simulink model "case5"  (R2024b)
settings: Solver=FixedStepAuto  StartTime=0  StopTime=1  FixedStep=1e-7  RelTol=1e-3
values from neighbouring files (symbols this model uses):
  SG_D_1_D = 0.01056    [IEEE9_case_parameters.m]    (also in case1_parameters.m; case2_parameters.m; case3_parameters.m; case4_parameters.m)
  SG_D_1_EnableSaturation = 0    [IEEE9_case_parameters.m]    (also in case1_parameters.m; case2_parameters.m; case3_parameters.m; case4_parameters.m)
  SG_D_1_f0 = 60    [IEEE9_case_parameters.m]    (also in case1_parameters.m; case2_parameters.m; case3_parameters.m; case4_parameters.m)
  SG_D_1_H = 7.5    [IEEE9_case_parameters.m]    (also in case1_parameters.m; case2_parameters.m; case3_parameters.m; case4_parameters.m)
  SG_D_1_K_A = 20    [IEEE9_case_parameters.m]    (also in case1_parameters.m; case2_parameters.m; case3_parameters.m; case4_parameters.m)
  SG_D_1_K_E = 1.000000e+1    (= 10)    [IEEE9_case_parameters.m]    (also in case1_parameters.m; case2_parameters.m; case3_parameters.m; case4_parameters.m)
  SG_D_1_K_F = 2.363    [IEEE9_case_parameters.m]    (also in case1_parameters.m; case2_parameters.m; case3_parameters.m; case4_parameters.m)
  SG_D_1_K_s = 0.5    [IEEE9_case_parameters.m]    (also in case1_parameters.m = 5; case2_parameters.m = 5; case3_parameters.m = 5; case4_parameters.m = 5)
  SG_D_1_R_a = 0.001088    [IEEE9_case_parameters.m]    (also in case1_parameters.m; case2_parameters.m; case3_parameters.m; case4_parameters.m)
  SG_D_1_S_A = 1    [IEEE9_case_parameters.m]    (also in case1_parameters.m; case2_parameters.m; case3_parameters.m; case4_parameters.m)
  SG_D_1_S_B = 0.103    [IEEE9_case_parameters.m]    (also in case1_parameters.m; case2_parameters.m; case3_parameters.m; case4_parameters.m)
  SG_D_1_S_N = 10.659857    [IEEE9_case_parameters.m]    (also in case1_parameters.m; case2_parameters.m; case3_parameters.m; case4_parameters.m)
  SG_D_1_SpeedPara = 200    [IEEE9_case_parameters.m]    (also in case1_parameters.m; case2_parameters.m; case3_parameters.m; case4_parameters.m)
  SG_D_1_T_0 = 0.720173    [IEEE9_case_parameters.m]    (also in case1_parameters.m = 0.755522; case2_parameters.m = 0.808931; case3_parameters.m = 0.869402; case4_parameters.m = 0.729316)
  SG_D_1_T_1 = 0.3    [IEEE9_case_parameters.m]    (also in case1_parameters.m; case2_parameters.m; case3_parameters.m; case4_parameters.m)
  SG_D_1_T_2 = 0.05    [IEEE9_case_parameters.m]    (also in case1_parameters.m; case2_parameters.m; case3_parameters.m; case4_parameters.m)
  SG_D_1_T_3 = 0.02    [IEEE9_case_parameters.m]    (also in case1_parameters.m; case2_parameters.m; case3_parameters.m; case4_parameters.m)
  SG_D_1_T_4 = 0.005    [IEEE9_case_parameters.m]    (also in case1_parameters.m; case2_parameters.m; case3_parameters.m; case4_parameters.m)
  SG_D_1_T_A = 0.02    [IEEE9_case_parameters.m]    (also in case1_parameters.m; case2_parameters.m; case3_parameters.m; case4_parameters.m)
  SG_D_1_T_dd = 8.000000e+0    (= 8)    [IEEE9_case_parameters.m]    (also in case1_parameters.m; case2_parameters.m; case3_parameters.m; case4_parameters.m)
  SG_D_1_T_ddd = 0.04    [IEEE9_case_parameters.m]    (also in case1_parameters.m; case2_parameters.m; case3_parameters.m; case4_parameters.m)
  SG_D_1_T_E = 0.314    [IEEE9_case_parameters.m]    (also in case1_parameters.m; case2_parameters.m; case3_parameters.m; case4_parameters.m)
  SG_D_1_T_F = 0.35    [IEEE9_case_parameters.m]    (also in case1_parameters.m; case2_parameters.m; case3_parameters.m; case4_parameters.m)
  SG_D_1_T_qd = 0.8    [IEEE9_case_parameters.m]    (also in case1_parameters.m; case2_parameters.m; case3_parameters.m; case4_parameters.m)
  SG_D_1_T_qdd = 0.02    [IEEE9_case_parameters.m]    (also in case1_parameters.m; case2_parameters.m; case3_parameters.m; case4_parameters.m)
  SG_D_1_T_speed = 0.1    [IEEE9_case_parameters.m]    (also in case1_parameters.m = 200; case2_parameters.m = 200; case3_parameters.m = 200; case4_parameters.m = 200)
  SG_D_1_T_w = 0.5    [IEEE9_case_parameters.m]    (also in case1_parameters.m; case2_parameters.m; case3_parameters.m; case4_parameters.m)
  SG_D_1_V_ref = 1.990276    [IEEE9_case_parameters.m]    (also in case1_parameters.m = 2.042296; case2_parameters.m = 2.051388; case3_parameters.m = 2.089584; case4_parameters.m = 2.01845)
  SG_D_1_w_ref = 376.991118    [IEEE9_case_parameters.m]    (also in case1_parameters.m; case2_parameters.m; case3_parameters.m; case4_parameters.m)
  SG_D_1_wb = 6.000000e+1    (= 60)    [IEEE9_case_parameters.m]    (also in case1_parameters.m; case2_parameters.m; case3_parameters.m; case4_parameters.m)
  SG_D_1_x_d = 1.9    [IEEE9_case_parameters.m]    (also in case1_parameters.m; case2_parameters.m; case3_parameters.m; case4_parameters.m)
  SG_D_1_x_dd = 0.302    [IEEE9_case_parameters.m]    (also in case1_parameters.m; case2_parameters.m; case3_parameters.m; case4_parameters.m)
  SG_D_1_x_ddd = 0.204    [IEEE9_case_parameters.m]    (also in case1_parameters.m; case2_parameters.m; case3_parameters.m; case4_parameters.m)
  SG_D_1_x_l = 0.05    [IEEE9_case_parameters.m]    (also in case1_parameters.m; case2_parameters.m; case3_parameters.m; case4_parameters.m)
  SG_D_1_x_q = 1.3    [IEEE9_case_parameters.m]    (also in case1_parameters.m; case2_parameters.m; case3_parameters.m; case4_parameters.m)
  SG_D_1_x_qd = 0.5    [IEEE9_case_parameters.m]    (also in case1_parameters.m; case2_parameters.m; case3_parameters.m; case4_parameters.m)
  SG_D_1_x_qdd = 0.3    [IEEE9_case_parameters.m]    (also in case1_parameters.m; case2_parameters.m; case3_parameters.m; case4_parameters.m)
  SG_D_2_D = 0.02    [IEEE9_case_parameters.m]    (also in case1_parameters.m; case2_parameters.m; case3_parameters.m; case4_parameters.m)
  SG_D_2_EnableSaturation = 0    [IEEE9_case_parameters.m]    (also in case1_parameters.m; case2_parameters.m; case3_parameters.m; case4_parameters.m)
  SG_D_2_f0 = 60    [IEEE9_case_parameters.m]    (also in case1_parameters.m; case2_parameters.m; case3_parameters.m; case4_parameters.m)
  SG_D_2_H = 8.000000e+0    (= 8)    [IEEE9_case_parameters.m]    (also in case1_parameters.m; case2_parameters.m; case3_parameters.m; case4_parameters.m)
  SG_D_2_K_A = 20    [IEEE9_case_parameters.m]    (also in case1_parameters.m; case2_parameters.m; case3_parameters.m; case4_parameters.m)
  SG_D_2_K_E = 1.000000e+1    (= 10)    [IEEE9_case_parameters.m]    (also in case1_parameters.m; case2_parameters.m; case3_parameters.m; case4_parameters.m)
  SG_D_2_K_F = 2.363    [IEEE9_case_parameters.m]    (also in case1_parameters.m; case2_parameters.m; case3_parameters.m; case4_parameters.m)
  SG_D_2_K_s = 0.5    [IEEE9_case_parameters.m]    (also in case1_parameters.m = 4; case2_parameters.m = 4; case3_parameters.m = 4; case4_parameters.m = 4)
  SG_D_2_R_a = 0.001088    [IEEE9_case_parameters.m]    (also in case1_parameters.m; case2_parameters.m; case3_parameters.m; case4_parameters.m)
  SG_D_2_S_A = 1    [IEEE9_case_parameters.m]    (also in case1_parameters.m; case2_parameters.m; case3_parameters.m; case4_parameters.m)
  SG_D_2_S_B = 0.103    [IEEE9_case_parameters.m]    (also in case1_parameters.m; case2_parameters.m; case3_parameters.m; case4_parameters.m)
  SG_D_2_S_N = 10.659857    [IEEE9_case_parameters.m]    (also in case1_parameters.m; case2_parameters.m; case3_parameters.m; case4_parameters.m)
  SG_D_2_SpeedPara = 200    [IEEE9_case_parameters.m]    (also in case1_parameters.m; case2_parameters.m; case3_parameters.m; case4_parameters.m)
  SG_D_2_T_0 = 1.632913    [IEEE9_case_parameters.m]    (also in case1_parameters.m = 1.632925; case2_parameters.m = 1.632915; case3_parameters.m = 1.632914; case4_parameters.m = 1.632927)
  SG_D_2_T_1 = 0.2    [IEEE9_case_parameters.m]    (also in case1_parameters.m; case2_parameters.m; case3_parameters.m; case4_parameters.m)
  SG_D_2_T_2 = 0.05    [IEEE9_case_parameters.m]    (also in case1_parameters.m; case2_parameters.m; case3_parameters.m; case4_parameters.m)
  SG_D_2_T_3 = 0.02    [IEEE9_case_parameters.m]    (also in case1_parameters.m; case2_parameters.m; case3_parameters.m; case4_parameters.m)
  SG_D_2_T_4 = 0.005    [IEEE9_case_parameters.m]    (also in case1_parameters.m; case2_parameters.m; case3_parameters.m; case4_parameters.m)
  SG_D_2_T_A = 0.02    [IEEE9_case_parameters.m]    (also in case1_parameters.m; case2_parameters.m; case3_parameters.m; case4_parameters.m)
  SG_D_2_T_dd = 7.9    [IEEE9_case_parameters.m]    (also in case1_parameters.m; case2_parameters.m; case3_parameters.m; case4_parameters.m)
  SG_D_2_T_ddd = 0.04    [IEEE9_case_parameters.m]    (also in case1_parameters.m; case2_parameters.m; case3_parameters.m; case4_parameters.m)
  SG_D_2_T_E = 0.314    [IEEE9_case_parameters.m]    (also in case1_parameters.m; case2_parameters.m; case3_parameters.m; case4_parameters.m)
  SG_D_2_T_F = 0.35    [IEEE9_case_parameters.m]    (also in case1_parameters.m; case2_parameters.m; case3_parameters.m; case4_parameters.m)
  SG_D_2_T_qd = 0.8    [IEEE9_case_parameters.m]    (also in case1_parameters.m; case2_parameters.m; case3_parameters.m; case4_parameters.m)
  SG_D_2_T_qdd = 0.015    [IEEE9_case_parameters.m]    (also in case1_parameters.m; case2_parameters.m; case3_parameters.m; case4_parameters.m)
  SG_D_2_T_speed = 0.1    [IEEE9_case_parameters.m]    (also in case1_parameters.m = 150; case2_parameters.m = 150; case3_parameters.m = 150; case4_parameters.m = 150)
  SG_D_2_T_w = 0.35    [IEEE9_case_parameters.m]    (also in case1_parameters.m; case2_parameters.m; case3_parameters.m; case4_parameters.m)
  SG_D_2_V_ref = 2.58547    [IEEE9_case_parameters.m]    (also in case1_parameters.m = 2.597896; case2_parameters.m = 2.587136; case3_parameters.m = 2.586042; case4_parameters.m = 2.599679)
  SG_D_2_w_ref = 376.991118    [IEEE9_case_parameters.m]    (also in case1_parameters.m; case2_parameters.m; case3_parameters.m; case4_parameters.m)
  SG_D_2_wb = 6.000000e+1    (= 60)    [IEEE9_case_parameters.m]    (also in case1_parameters.m; case2_parameters.m; case3_parameters.m; case4_parameters.m)
  SG_D_2_x_d = 1.8    [IEEE9_case_parameters.m]    (also in case1_parameters.m; case2_parameters.m; case3_parameters.m; case4_parameters.m)
  SG_D_2_x_dd = 0.302    [IEEE9_case_parameters.m]    (also in case1_parameters.m; case2_parameters.m; case3_parameters.m; case4_parameters.m)
  SG_D_2_x_ddd = 0.204    [IEEE9_case_parameters.m]    (also in case1_parameters.m; case2_parameters.m; case3_parameters.m; case4_parameters.m)
  SG_D_2_x_l = 0.05    [IEEE9_case_parameters.m]    (also in case1_parameters.m; case2_parameters.m; case3_parameters.m; case4_parameters.m)
  SG_D_2_x_q = 1.25    [IEEE9_case_parameters.m]    (also in case1_parameters.m; case2_parameters.m; case3_parameters.m; case4_parameters.m)
  SG_D_2_x_qd = 0.5    [IEEE9_case_parameters.m]    (also in case1_parameters.m; case2_parameters.m; case3_parameters.m; case4_parameters.m)
  SG_D_2_x_qdd = 0.3    [IEEE9_case_parameters.m]    (also in case1_parameters.m; case2_parameters.m; case3_parameters.m; case4_parameters.m)
  SG_D_3_D = 0.02    [IEEE9_case_parameters.m]    (also in case1_parameters.m; case2_parameters.m; case3_parameters.m; case4_parameters.m)
  SG_D_3_EnableSaturation = 0    [IEEE9_case_parameters.m]    (also in case1_parameters.m; case2_parameters.m; case3_parameters.m; case4_parameters.m)
  SG_D_3_f0 = 60    [IEEE9_case_parameters.m]    (also in case1_parameters.m; case2_parameters.m; case3_parameters.m; case4_parameters.m)
  SG_D_3_H = 7.7    [IEEE9_case_parameters.m]    (also in case1_parameters.m; case2_parameters.m; case3_parameters.m; case4_parameters.m)
  SG_D_3_K_A = 20    [IEEE9_case_parameters.m]    (also in case1_parameters.m; case2_parameters.m; case3_parameters.m; case4_parameters.m)
  SG_D_3_K_E = 1.000000e+1    (= 10)    [IEEE9_case_parameters.m]    (also in case1_parameters.m; case2_parameters.m; case3_parameters.m; case4_parameters.m)
  SG_D_3_K_F = 2.363    [IEEE9_case_parameters.m]    (also in case1_parameters.m; case2_parameters.m; case3_parameters.m; case4_parameters.m)
  SG_D_3_K_s = 0.2    [IEEE9_case_parameters.m]    (also in case1_parameters.m = 2; case2_parameters.m = 2; case3_parameters.m = 2; case4_parameters.m = 2)
  SG_D_3_R_a = 0.001088    [IEEE9_case_parameters.m]    (also in case1_parameters.m; case2_parameters.m; case3_parameters.m; case4_parameters.m)
  SG_D_3_S_A = 1    [IEEE9_case_parameters.m]    (also in case1_parameters.m; case2_parameters.m; case3_parameters.m; case4_parameters.m)
  SG_D_3_S_B = 0.103    [IEEE9_case_parameters.m]    (also in case1_parameters.m; case2_parameters.m; case3_parameters.m; case4_parameters.m)
  SG_D_3_S_N = 10.659857    [IEEE9_case_parameters.m]    (also in case1_parameters.m; case2_parameters.m; case3_parameters.m; case4_parameters.m)
  SG_D_3_SpeedPara = 200    [IEEE9_case_parameters.m]    (also in case1_parameters.m; case2_parameters.m; case3_parameters.m; case4_parameters.m)
  SG_D_3_T_0 = 0.850788    [IEEE9_case_parameters.m]    (also in case1_parameters.m = 0.850786; case2_parameters.m = 0.850787; case3_parameters.m; case4_parameters.m = 0.850786)
  SG_D_3_T_1 = 0.2    [IEEE9_case_parameters.m]    (also in case1_parameters.m; case2_parameters.m; case3_parameters.m; case4_parameters.m)
  SG_D_3_T_2 = 0.05    [IEEE9_case_parameters.m]    (also in case1_parameters.m; case2_parameters.m; case3_parameters.m; case4_parameters.m)
  SG_D_3_T_3 = 0.02    [IEEE9_case_parameters.m]    (also in case1_parameters.m; case2_parameters.m; case3_parameters.m; case4_parameters.m)
  SG_D_3_T_4 = 0.005    [IEEE9_case_parameters.m]    (also in case1_parameters.m; case2_parameters.m; case3_parameters.m; case4_parameters.m)
  SG_D_3_T_A = 0.02    [IEEE9_case_parameters.m]    (also in case1_parameters.m; case2_parameters.m; case3_parameters.m; case4_parameters.m)
  SG_D_3_T_dd = 8.1    [IEEE9_case_parameters.m]    (also in case1_parameters.m; case2_parameters.m; case3_parameters.m; case4_parameters.m)
  SG_D_3_T_ddd = 0.04    [IEEE9_case_parameters.m]    (also in case1_parameters.m; case2_parameters.m; case3_parameters.m; case4_parameters.m)
  SG_D_3_T_E = 0.314    [IEEE9_case_parameters.m]    (also in case1_parameters.m; case2_parameters.m; case3_parameters.m; case4_parameters.m)
  SG_D_3_T_F = 0.35    [IEEE9_case_parameters.m]    (also in case1_parameters.m; case2_parameters.m; case3_parameters.m; case4_parameters.m)
  SG_D_3_T_qd = 0.8    [IEEE9_case_parameters.m]    (also in case1_parameters.m; case2_parameters.m; case3_parameters.m; case4_parameters.m)
  SG_D_3_T_qdd = 0.015    [IEEE9_case_parameters.m]    (also in case1_parameters.m; case2_parameters.m; case3_parameters.m; case4_parameters.m)
  SG_D_3_T_speed = 0.1    [IEEE9_case_parameters.m]    (also in case1_parameters.m = 180; case2_parameters.m = 180; case3_parameters.m = 180; case4_parameters.m = 180)
  SG_D_3_T_w = 0.4    [IEEE9_case_parameters.m]    (also in case1_parameters.m; case2_parameters.m; case3_parameters.m; case4_parameters.m)
  SG_D_3_V_ref = 1.892727    [IEEE9_case_parameters.m]    (also in case1_parameters.m = 1.906439; case2_parameters.m = 1.895535; case3_parameters.m = 1.892105; case4_parameters.m = 1.906598)
  SG_D_3_w_ref = 376.991118    [IEEE9_case_parameters.m]    (also in case1_parameters.m; case2_parameters.m; case3_parameters.m; case4_parameters.m)
  SG_D_3_wb = 6.000000e+1    (= 60)    [IEEE9_case_parameters.m]    (also in case1_parameters.m; case2_parameters.m; case3_parameters.m; case4_parameters.m)
  SG_D_3_x_d = 1.85    [IEEE9_case_parameters.m]    (also in case1_parameters.m; case2_parameters.m; case3_parameters.m; case4_parameters.m)
  SG_D_3_x_dd = 0.302    [IEEE9_case_parameters.m]    (also in case1_parameters.m; case2_parameters.m; case3_parameters.m; case4_parameters.m)
  SG_D_3_x_ddd = 0.204    [IEEE9_case_parameters.m]    (also in case1_parameters.m; case2_parameters.m; case3_parameters.m; case4_parameters.m)
  SG_D_3_x_l = 0.05    [IEEE9_case_parameters.m]    (also in case1_parameters.m; case2_parameters.m; case3_parameters.m; case4_parameters.m)
  SG_D_3_x_q = 1.2    [IEEE9_case_parameters.m]    (also in case1_parameters.m; case2_parameters.m; case3_parameters.m; case4_parameters.m)
  SG_D_3_x_qd = 0.5    [IEEE9_case_parameters.m]    (also in case1_parameters.m; case2_parameters.m; case3_parameters.m; case4_parameters.m)
  SG_D_3_x_qdd = 0.3    [IEEE9_case_parameters.m]    (also in case1_parameters.m; case2_parameters.m; case3_parameters.m; case4_parameters.m)
(part 5 of 12)

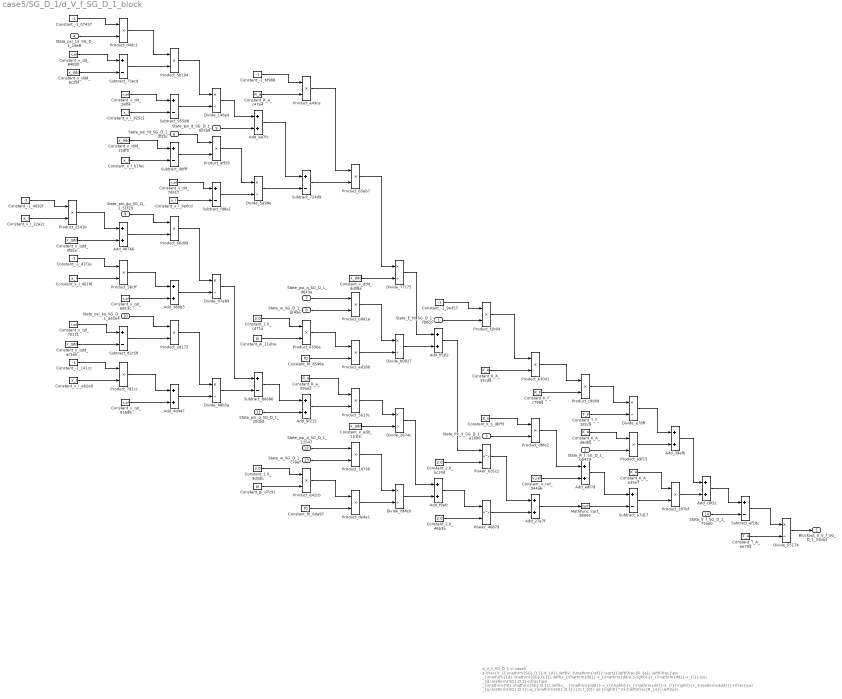
== system case5/SG_D_1/d_V_f_SG_D_1_block ==
  note: d_V_f_SG_D_1 in case5
      | $-\frac{V_{f,\mathrm{SG},D,1}-K_{A}\,\left(V_{\mathrm{ref}}-\sqrt{{\left(\frac{R_{a}\,\left(\frac{\psi _{\mathrm{1d},\mathrm{SG},D,1}\,\left(x_{\mathrm{dd}}-x_{\mathrm{ddd}}\right)}{x_{\mathrm{dd}}-x_{l}}-\psi _{d,\mathrm{SG},D,1}+\frac{\psi _{\mathrm{fd},\mathrm{SG},D,1}\,\left(x_{\mathrm{ddd}}-x_{l}\right)}{x_{\mathrm{dd}}-x_{l}}\right)}{x_{\mathrm{ddd}}}+\frac{\psi _{q,\mathrm{SG},D,1}\,w_{\mathrm{SG},D,1}}{2\,f_{0}\,\pi }\right)}^2+{\left(\frac{R_{a}\,\left(\psi _{q,\mathrm{SG},D,1}+\frac{\psi _{\mathrm{gq},\mathrm{SG},D,1}\,\left(x_{l}-x_{\mathrm{qdd}}\right)}{x_{l}-x_{\mathrm{qd}}}+\frac{\psi _{\mathrm{kq},\mathrm{SG},D,1}\,\left(x_{\mathrm{qd}}-x_{\mathrm{qdd}}\right)}{x_{l}-x_{\mathrm{qd}}}\right)}{x_{\mathrm{qdd}}}+\frac{\psi _{d,\mathrm{SG},D,1}\,w_{\mathrm{SG},D,1}}{2\,f_{0}\,\pi }\right)}^2}+K_{s}\,\mathrm{Px}_{3,\mathrm{SG},D,1}\right)-K_{A}\,R_{f,\mathrm{SG},D,1}+\frac{E_{\mathrm{fd},\mathrm{SG},D,1}\,K_{A}\,K_{F}}{T_{F}}}{T_{A}}$
      | Automatically generated on 2025-10-31 19:10:20 .
  State_E_fd_SG_D_1_f00c0 : Inport
  State_R_f_SG_D_1_bb479 : Inport  Port=2
  State_Px_3_SG_D_1_a16d6 : Inport  Port=3
  State_psi_1d_SG_D_1_19aff : Inport  Port=4
  State_psi_d_SG_D_1_925b9 : Inport  Port=5
  State_psi_fd_SG_D_1_3f25c : Inport  Port=6
  State_psi_q_SG_D_1_d643a : Inport  Port=7
  State_w_SG_D_1_bf45e : Inport  Port=8
  State_psi_gq_SG_D_1_51f29 : Inport  Port=9
  State_psi_kq_SG_D_1_ae2e4 : Inport  Port=10
  State_psi_q_SG_D_1_20da0 : Inport  Port=11
  State_psi_d_SG_D_1_12547 : Inport  Port=12
  State_w_SG_D_1_c7aef : Inport  Port=13
  State_V_f_SG_D_1_75aeb : Inport  Port=14
  Add_27e7f : Sum
  Add_380b3 : Sum
  Add_39efb : Sum
  Add_40766 : Sum
  Add_4d447 : Sum
  Add_9f215 : Sum
  Add_adf7d : Sum
  Add_ba7fc : Sum
  Add_c8f2c : Sum
  Add_f9afc : Sum
  Add_ff182 : Sum
  Constant_-1_07437 : Constant  Value=-1
  Constant_-1_141cc : Constant  Value=-1
  Constant_-1_4092f : Constant  Value=-1
  Constant_-1_6f988 : Constant  Value=-1
  Constant_-1_9a357 : Constant  Value=-1
  Constant_-1_d1f1e : Constant  Value=-1
  Constant_2.0_46b3a : Constant  Value=2.0
  Constant_2.0_9d3db : Constant  Value=2.0
  Constant_2.0_bc20d : Constant  Value=2.0
  Constant_2.0_cd71a : Constant  Value=2.0
  Constant_K_A_35cd9 : Constant  Value=K_A
  Constant_K_A_a35e7 : Constant  Value=K_A
  Constant_K_A_d6db0 : Constant  Value=K_A
  Constant_K_F_c798d : Constant  Value=K_F
  Constant_K_s_dbff3 : Constant  Value=K_s
  Constant_R_a_09ae2 : Constant  Value=R_a
  Constant_R_a_c47e4 : Constant  Value=R_a
  Constant_T_A_ee70d : Constant  Value=T_A
  Constant_T_F_181c9 : Constant  Value=T_F
  Constant_V_ref_044a6 : Constant  Value=V_ref
  Constant_f0_6da97 : Constant  Value=f0
  Constant_f0_8546e : Constant  Value=f0
  Constant_pi_11eba : Constant  Value=pi
  Constant_pi_d7c91 : Constant  Value=pi
  Constant_x_dd_26ff4 : Constant  Value=x_dd
  Constant_x_dd_7d917 : Constant  Value=x_dd
  Constant_x_dd_84830 : Constant  Value=x_dd
  Constant_x_ddd_218f0 : Constant  Value=x_ddd
  Constant_x_ddd_8c29f : Constant  Value=x_ddd
  Constant_x_ddd_dd08a : Constant  Value=x_ddd
  Constant_x_l_22a2c : Constant  Value=x_l
  Constant_x_l_401f6 : Constant  Value=x_l
  Constant_x_l_925c1 : Constant  Value=x_l
  Constant_x_l_9e0cd : Constant  Value=x_l
  Constant_x_l_b1fec : Constant  Value=x_l
  Constant_x_l_eb2e9 : Constant  Value=x_l
  Constant_x_qd_6813c : Constant  Value=x_qd
  Constant_x_qd_91b86 : Constant  Value=x_qd
  Constant_x_qd_f0131 : Constant  Value=x_qd
  Constant_x_qdd_151fe : Constant  Value=x_qdd
  Constant_x_qdd_3f8ce : Constant  Value=x_qdd
  Constant_x_qdd_ac5ab : Constant  Value=x_qdd
  Divide_07e89 : Product  Inputs=*/
  Divide_146e4 : Product  Inputs=*/
  Divide_2674c : Product  Inputs=*/
  Divide_55174 : Product  Inputs=*/
  Divide_5a98e : Product  Inputs=*/
  Divide_77c75 : Product  Inputs=*/
  Divide_86fe9 : Product  Inputs=*/
  Divide_b0027 : Product  Inputs=*/
  Divide_b8b5a : Product  Inputs=*/
  Divide_e78ff : Product  Inputs=*/
  MathFunc_sqrt_85061 : Sqrt
  Power_46879 : Math  Operator=pow
  Power_b31c2 : Math  Operator=pow
  Product_14736 : Product
  Product_2541b : Product
  Product_297bf : Product
  Product_2d172 : Product
  Product_5613c : Product
  Product_56cff : Product
  Product_5b104 : Product
  Product_633ba : Product
  Product_65eb7 : Product
  Product_66d09 : Product
  Product_7d1cc : Product
  Product_a49ce : Product
  Product_a9f15 : Product
  Product_ad180 : Product
  Product_aff29 : Product
  Product_b3041 : Product
  Product_b8d1a : Product
  Product_c9909 : Product
  Product_d4dc1 : Product
  Product_dbfe2 : Product
  Product_de4e1 : Product
  Product_e42cb : Product
  Product_f2b04 : Product
  Subtract_724d9 : Sum  Inputs=+-
  Subtract_73acd : Sum  Inputs=+-
  Subtract_80686 : Sum  Inputs=+-
  Subtract_95588 : Sum  Inputs=+-
  Subtract_a7d17 : Sum  Inputs=+-
  Subtract_d0fff : Sum  Inputs=+-
  Subtract_d2c58 : Sum  Inputs=+-
  Subtract_ef18c : Sum  Inputs=+-
  Subtract_fd8a1 : Sum  Inputs=+-
  Blockout_d_V_f_SG_D_1_31ba3 : Outport
  wires:
  Constant_-1_141cc/1 -> Product_7d1cc/1
  Constant_-1_4092f/1 -> Product_2541b/1
  State_psi_d_SG_D_1_12547/1 -> Product_14736/1
  Constant_x_qd_91b86/1 -> Add_4d447/2
  Constant_x_qdd_3f8ce/1 -> Add_40766/2
  State_w_SG_D_1_c7aef/1 -> Product_14736/2
  Constant_x_l_22a2c/1 -> Product_2541b/2
  Subtract_724d9/1 -> Product_65eb7/2
  Constant_x_l_eb2e9/1 -> Product_7d1cc/2
  Constant_x_dd_84830/1 -> Subtract_73acd/1
  Constant_R_a_c47e4/1 -> Product_a49ce/2
  Constant_-1_07437/1 -> Product_d4dc1/1
  Divide_5a98e/1 -> Subtract_724d9/2
  Constant_x_ddd_8c29f/1 -> Subtract_73acd/2
  Add_4d447/1 -> Divide_b8b5a/2
  State_psi_1d_SG_D_1_19aff/1 -> Product_d4dc1/2
  Add_380b3/1 -> Divide_07e89/2
  Subtract_d2c58/1 -> Product_2d172/2
  Product_c9909/1 -> Divide_e78ff/1
  Product_633ba/1 -> Product_ad180/1
  Product_2541b/1 -> Add_40766/1
  Constant_-1_d1f1e/1 -> Product_56cff/1
  Constant_x_l_401f6/1 -> Product_56cff/2
  Add_ba7fc/1 -> Subtract_724d9/1
  Constant_2.0_9d3db/1 -> Product_e42cb/1
  Constant_x_qd_f0131/1 -> Subtract_d2c58/1
  Product_d4dc1/1 -> Product_5b104/1
  Constant_pi_d7c91/1 -> Product_e42cb/2
  Constant_x_qdd_ac5ab/1 -> Subtract_d2c58/2
  Subtract_73acd/1 -> Product_5b104/2
  State_psi_q_SG_D_1_20da0/1 -> Add_9f215/2
  Constant_x_dd_26ff4/1 -> Subtract_95588/1
  Constant_x_l_925c1/1 -> Subtract_95588/2
  Constant_x_ddd_218f0/1 -> Subtract_d0fff/1
  Constant_x_l_b1fec/1 -> Subtract_d0fff/2
  State_psi_gq_SG_D_1_51f29/1 -> Product_66d09/1
  Add_40766/1 -> Product_66d09/2
  Product_56cff/1 -> Add_380b3/1
  Constant_x_qd_6813c/1 -> Add_380b3/2
  Divide_146e4/1 -> Add_ba7fc/1
  Subtract_95588/1 -> Divide_146e4/2
  State_psi_kq_SG_D_1_ae2e4/1 -> Product_2d172/1
  Divide_55174/1 -> Blockout_d_V_f_SG_D_1_31ba3/1
  Product_7d1cc/1 -> Add_4d447/1
  Product_5b104/1 -> Divide_146e4/1
  State_psi_fd_SG_D_1_3f25c/1 -> Product_aff29/1
  State_w_SG_D_1_bf45e/1 -> Product_b8d1a/2
  Subtract_d0fff/1 -> Product_aff29/2
  Constant_x_dd_7d917/1 -> Subtract_fd8a1/1
  Constant_x_l_9e0cd/1 -> Subtract_fd8a1/2
  Product_66d09/1 -> Divide_07e89/1
  Product_a49ce/1 -> Product_65eb7/1
  Product_2d172/1 -> Divide_b8b5a/1
  State_psi_d_SG_D_1_925b9/1 -> Add_ba7fc/2
  Product_aff29/1 -> Divide_5a98e/1
  Subtract_fd8a1/1 -> Divide_5a98e/2
  Divide_07e89/1 -> Subtract_80686/1
  Divide_b8b5a/1 -> Subtract_80686/2
  Constant_-1_6f988/1 -> Product_a49ce/1
  Constant_2.0_cd71a/1 -> Product_633ba/1
  Constant_pi_11eba/1 -> Product_633ba/2
  Subtract_80686/1 -> Add_9f215/1
  State_psi_q_SG_D_1_d643a/1 -> Product_b8d1a/1
  Constant_f0_8546e/1 -> Product_ad180/2
  Constant_R_a_09ae2/1 -> Product_5613c/1
  Add_9f215/1 -> Product_5613c/2
  Product_e42cb/1 -> Product_de4e1/1
  Power_b31c2/1 -> Add_27e7f/1
  Constant_f0_6da97/1 -> Product_de4e1/2
  Product_65eb7/1 -> Divide_77c75/1
  Constant_x_ddd_dd08a/1 -> Divide_77c75/2
  Product_b8d1a/1 -> Divide_b0027/1
  Product_ad180/1 -> Divide_b0027/2
  Product_5613c/1 -> Divide_2674c/1
  Constant_x_qdd_151fe/1 -> Divide_2674c/2
  Product_14736/1 -> Divide_86fe9/1
  Product_de4e1/1 -> Divide_86fe9/2
  Divide_77c75/1 -> Add_ff182/1
  Divide_b0027/1 -> Add_ff182/2
  Divide_2674c/1 -> Add_f9afc/1
  Divide_86fe9/1 -> Add_f9afc/2
  Constant_-1_9a357/1 -> Product_f2b04/1
  State_E_fd_SG_D_1_f00c0/1 -> Product_f2b04/2
  Add_ff182/1 -> Power_b31c2/1
  Constant_2.0_bc20d/1 -> Power_b31c2/2
  Add_f9afc/1 -> Power_46879/1
  Constant_2.0_46b3a/1 -> Power_46879/2
  Product_f2b04/1 -> Product_b3041/1
  Constant_K_A_35cd9/1 -> Product_b3041/2
  Constant_K_s_dbff3/1 -> Product_dbfe2/1
  State_Px_3_SG_D_1_a16d6/1 -> Product_dbfe2/2
  Power_46879/1 -> Add_27e7f/2
  Divide_e78ff/1 -> Add_39efb/1
  Product_b3041/1 -> Product_c9909/1
  Constant_K_F_c798d/1 -> Product_c9909/2
  Product_dbfe2/1 -> Add_adf7d/1
  Constant_V_ref_044a6/1 -> Add_adf7d/2
  Add_27e7f/1 -> MathFunc_sqrt_85061/1
  Constant_T_F_181c9/1 -> Divide_e78ff/2
  Constant_K_A_d6db0/1 -> Product_a9f15/1
  State_R_f_SG_D_1_bb479/1 -> Product_a9f15/2
  Add_adf7d/1 -> Subtract_a7d17/1
  MathFunc_sqrt_85061/1 -> Subtract_a7d17/2
  Constant_T_A_ee70d/1 -> Divide_55174/2
  Product_a9f15/1 -> Add_39efb/2
  Constant_K_A_a35e7/1 -> Product_297bf/1
  Subtract_a7d17/1 -> Product_297bf/2
  Add_39efb/1 -> Add_c8f2c/1
  Product_297bf/1 -> Add_c8f2c/2
  Add_c8f2c/1 -> Subtract_ef18c/1
  State_V_f_SG_D_1_75aeb/1 -> Subtract_ef18c/2
  Subtract_ef18c/1 -> Divide_55174/1

== system case5/SG_D_1/d_psi_1d_SG_D_1_block ==
  note: d_psi_1d_SG_D_1 in case5
      | $-\frac{\psi _{\mathrm{1d},\mathrm{SG},D,1}-\psi _{\mathrm{fd},\mathrm{SG},D,1}+\frac{\left(x_{\mathrm{dd}}-x_{l}\right)\,\left(\frac{\psi _{\mathrm{1d},\mathrm{SG},D,1}\,\left(x_{\mathrm{dd}}-x_{\mathrm{ddd}}\right)}{x_{\mathrm{dd}}-x_{l}}-\psi _{d,\mathrm{SG},D,1}+\frac{\psi _{\mathrm{fd},\mathrm{SG},D,1}\,\left(x_{\mathrm{ddd}}-x_{l}\right)}{x_{\mathrm{dd}}-x_{l}}\right)}{x_{\mathrm{ddd}}}}{T_{\mathrm{ddd}}}$
      | Automatically generated on 2025-10-31 19:09:54 .
  State_psi_1d_SG_D_1_12b31 : Inport
  State_psi_fd_SG_D_1_45ba0 : Inport  Port=2
  State_psi_1d_SG_D_1_6ec63 : Inport  Port=3
  State_psi_d_SG_D_1_0b6f3 : Inport  Port=4
  State_psi_fd_SG_D_1_34365 : Inport  Port=5
  Add_558c6 : Sum
  Add_b9c2c : Sum
  Add_da64c : Sum
  Constant_-1_5cb57 : Constant  Value=-1
  Constant_-1_78057 : Constant  Value=-1
  Constant_T_ddd_d6c90 : Constant  Value=T_ddd
  Constant_x_dd_5aee0 : Constant  Value=x_dd
  Constant_x_dd_6b9d0 : Constant  Value=x_dd
  Constant_x_dd_cb64c : Constant  Value=x_dd
  Constant_x_dd_e8196 : Constant  Value=x_dd
  Constant_x_ddd_347d4 : Constant  Value=x_ddd
  Constant_x_ddd_69ebe : Constant  Value=x_ddd
  Constant_x_ddd_d130c : Constant  Value=x_ddd
  Constant_x_l_15c3f : Constant  Value=x_l
  Constant_x_l_24a9a : Constant  Value=x_l
  Constant_x_l_61f26 : Constant  Value=x_l
  Constant_x_l_d01d0 : Constant  Value=x_l
  Divide_184a6 : Product  Inputs=*/
  Divide_1fbd8 : Product  Inputs=*/
  Divide_2731c : Product  Inputs=*/
  Divide_6e2e4 : Product  Inputs=*/
  Product_64b77 : Product
  Product_7d6d9 : Product
  Product_9126b : Product
  Product_caf0e : Product
  Product_f3d7c : Product
  Subtract_366dc : Sum  Inputs=+-
  Subtract_47175 : Sum  Inputs=+-
  Subtract_79194 : Sum  Inputs=+-
  Subtract_993eb : Sum  Inputs=+-
  Subtract_b4cc8 : Sum  Inputs=+-
  Subtract_ea900 : Sum  Inputs=+-
  Blockout_d_psi_1d_SG_D_1_a7c17 : Outport
  wires:
  Product_9126b/1 -> Product_64b77/1
  Constant_-1_78057/1 -> Product_9126b/1
  Subtract_47175/1 -> Product_64b77/2
  State_psi_1d_SG_D_1_6ec63/1 -> Product_9126b/2
  Subtract_366dc/1 -> Product_f3d7c/1
  State_psi_d_SG_D_1_0b6f3/1 -> Add_558c6/2
  Constant_x_dd_e8196/1 -> Subtract_b4cc8/1
  Constant_x_l_61f26/1 -> Subtract_366dc/2
  Constant_x_dd_5aee0/1 -> Subtract_47175/1
  Subtract_993eb/1 -> Product_caf0e/2
  Constant_x_l_24a9a/1 -> Subtract_b4cc8/2
  Divide_1fbd8/1 -> Subtract_ea900/2
  Constant_x_ddd_d130c/1 -> Subtract_47175/2
  Constant_x_ddd_347d4/1 -> Subtract_993eb/1
  Constant_x_l_15c3f/1 -> Subtract_993eb/2
  Add_da64c/1 -> Add_b9c2c/1
  Product_64b77/1 -> Divide_2731c/1
  Divide_184a6/1 -> Add_b9c2c/2
  Subtract_b4cc8/1 -> Divide_2731c/2
  State_psi_fd_SG_D_1_34365/1 -> Product_caf0e/1
  Constant_x_dd_6b9d0/1 -> Subtract_79194/1
  Constant_x_l_d01d0/1 -> Subtract_79194/2
  Constant_x_ddd_69ebe/1 -> Divide_184a6/2
  Subtract_ea900/1 -> Product_f3d7c/2
  Divide_2731c/1 -> Add_558c6/1
  Product_caf0e/1 -> Divide_1fbd8/1
  Subtract_79194/1 -> Divide_1fbd8/2
  Product_f3d7c/1 -> Divide_184a6/1
  Constant_x_dd_cb64c/1 -> Subtract_366dc/1
  Add_558c6/1 -> Subtract_ea900/1
  Constant_-1_5cb57/1 -> Product_7d6d9/1
  State_psi_1d_SG_D_1_12b31/1 -> Product_7d6d9/2
  Product_7d6d9/1 -> Add_da64c/1
  State_psi_fd_SG_D_1_45ba0/1 -> Add_da64c/2
  Add_b9c2c/1 -> Divide_6e2e4/1
  Constant_T_ddd_d6c90/1 -> Divide_6e2e4/2
  Divide_6e2e4/1 -> Blockout_d_psi_1d_SG_D_1_a7c17/1

== system case5/SG_D_1/d_psi_d_SG_D_1_block ==
  note: d_psi_d_SG_D_1 in case5
      | $2\,\pi \,f_{0}\,\left(v_{d,\mathrm{SG},D,1}\,\sin\left(\theta _{\mathrm{SG},D,1}\right)-v_{q,\mathrm{SG},D,1}\,\cos\left(\theta _{\mathrm{SG},D,1}\right)+\frac{R_{a}\,\left(\frac{\psi _{\mathrm{1d},\mathrm{SG},D,1}\,\left(x_{\mathrm{dd}}-x_{\mathrm{ddd}}\right)}{x_{\mathrm{dd}}-x_{l}}-\psi _{d,\mathrm{SG},D,1}+\frac{\psi _{\mathrm{fd},\mathrm{SG},D,1}\,\left(x_{\mathrm{ddd}}-x_{l}\right)}{x_{\mathrm{dd}}-x_{l}}\right)}{x_{\mathrm{ddd}}}+\frac{\psi _{q,\mathrm{SG},D,1}\,w_{\mathrm{SG},D,1}}{2\,f_{0}\,\pi }\right)$
      | Automatically generated on 2025-10-31 19:09:27 .
  State_psi_1d_SG_D_1_fda93 : Inport
  State_psi_d_SG_D_1_4a637 : Inport  Port=2
  State_psi_fd_SG_D_1_6a197 : Inport  Port=3
  Input_v_d_SG_D_1_eef26 : Inport  Port=4
  State_theta_SG_D_1_66e05 : Inport  Port=5
  Input_v_q_SG_D_1_363cd : Inport  Port=6
  State_theta_SG_D_1_b6b51 : Inport  Port=7
  State_psi_q_SG_D_1_30b1b : Inport  Port=8
  State_w_SG_D_1_1bb72 : Inport  Port=9
  Add_5e9fa : Sum
  Add_ba3bc : Sum
  Constant_-1_4fad5 : Constant  Value=-1
  Constant_-2.0_f3f6d : Constant  Value=-2.0
  Constant_2.0_44f7d : Constant  Value=2.0
  Constant_R_a_2f80d : Constant  Value=R_a
  Constant_f0_368b9 : Constant  Value=f0
  Constant_f0_e5b86 : Constant  Value=f0
  Constant_pi_be96d : Constant  Value=pi
  Constant_pi_f2e30 : Constant  Value=pi
  Constant_x_dd_58139 : Constant  Value=x_dd
  Constant_x_dd_b34e8 : Constant  Value=x_dd
  Constant_x_dd_ee10a : Constant  Value=x_dd
  Constant_x_ddd_46503 : Constant  Value=x_ddd
  Constant_x_ddd_8341f : Constant  Value=x_ddd
  Constant_x_ddd_bddcb : Constant  Value=x_ddd
  Constant_x_l_0d9cb : Constant  Value=x_l
  Constant_x_l_2646d : Constant  Value=x_l
  Constant_x_l_f167d : Constant  Value=x_l
  Divide_3c8e8 : Product  Inputs=*/
  Divide_da46f : Product  Inputs=*/
  Divide_e1c85 : Product  Inputs=*/
  Divide_f7e97 : Product  Inputs=*/
  MathFunc_cos_09e96 : Trigonometry  Operator=cos
  MathFunc_sin_1b65e : Trigonometry
  Product_0e1d5 : Product
  Product_12bd9 : Product
  Product_21a7d : Product
  Product_26a4a : Product
  Product_2eda6 : Product
  Product_3126e : Product
  Product_736ef : Product
  Product_8408d : Product
  Product_86144 : Product
  Product_9d7e6 : Product
  Product_dfb57 : Product
  Product_fa341 : Product
  Subtract_0a1d2 : Sum  Inputs=+-
  Subtract_2898f : Sum  Inputs=+-
  Subtract_309d5 : Sum  Inputs=+-
  Subtract_745a7 : Sum  Inputs=+-
  Subtract_b2c73 : Sum  Inputs=+-
  Subtract_c4249 : Sum  Inputs=+-
  Subtract_d41f1 : Sum  Inputs=+-
  Blockout_d_psi_d_SG_D_1_63859 : Outport
  wires:
  Add_5e9fa/1 -> Subtract_b2c73/1
  Product_8408d/1 -> Divide_da46f/1
  Subtract_c4249/1 -> Product_8408d/2
  Divide_da46f/1 -> Add_5e9fa/1
  Product_9d7e6/1 -> Product_8408d/1
  Constant_x_ddd_8341f/1 -> Subtract_c4249/2
  Constant_x_dd_b34e8/1 -> Subtract_c4249/1
  State_psi_1d_SG_D_1_fda93/1 -> Product_9d7e6/2
  Constant_-1_4fad5/1 -> Product_9d7e6/1
  Product_26a4a/1 -> Divide_f7e97/1
  Constant_x_l_f167d/1 -> Subtract_0a1d2/2
  State_psi_d_SG_D_1_4a637/1 -> Add_5e9fa/2
  Constant_x_dd_ee10a/1 -> Subtract_0a1d2/1
  Constant_x_ddd_bddcb/1 -> Subtract_d41f1/1
  Constant_x_l_2646d/1 -> Subtract_d41f1/2
  Subtract_0a1d2/1 -> Divide_da46f/2
  State_psi_fd_SG_D_1_6a197/1 -> Product_26a4a/1
  Constant_x_ddd_46503/1 -> Divide_e1c85/2
  Subtract_d41f1/1 -> Product_26a4a/2
  Product_21a7d/1 -> Subtract_2898f/2
  Constant_x_dd_58139/1 -> Subtract_309d5/1
  Constant_x_l_0d9cb/1 -> Subtract_309d5/2
  Subtract_309d5/1 -> Divide_f7e97/2
  Divide_f7e97/1 -> Subtract_b2c73/2
  Constant_R_a_2f80d/1 -> Product_3126e/1
  Subtract_b2c73/1 -> Product_3126e/2
  MathFunc_cos_09e96/1 -> Product_736ef/2
  State_theta_SG_D_1_66e05/1 -> MathFunc_sin_1b65e/1
  Divide_e1c85/1 -> Subtract_2898f/1
  Product_3126e/1 -> Divide_e1c85/1
  MathFunc_sin_1b65e/1 -> Product_21a7d/2
  Input_v_d_SG_D_1_eef26/1 -> Product_21a7d/1
  Product_86144/1 -> Blockout_d_psi_d_SG_D_1_63859/1
  Product_dfb57/1 -> Product_86144/1
  Product_2eda6/1 -> Product_dfb57/1
  State_theta_SG_D_1_b6b51/1 -> MathFunc_cos_09e96/1
  Constant_2.0_44f7d/1 -> Product_fa341/1
  Constant_pi_f2e30/1 -> Product_fa341/2
  Input_v_q_SG_D_1_363cd/1 -> Product_736ef/1
  Constant_f0_e5b86/1 -> Product_dfb57/2
  State_psi_q_SG_D_1_30b1b/1 -> Product_12bd9/1
  State_w_SG_D_1_1bb72/1 -> Product_12bd9/2
  Product_fa341/1 -> Product_0e1d5/1
  Constant_pi_be96d/1 -> Product_2eda6/2
  Constant_f0_368b9/1 -> Product_0e1d5/2
  Constant_-2.0_f3f6d/1 -> Product_2eda6/1
  Add_ba3bc/1 -> Subtract_745a7/1
  Subtract_2898f/1 -> Add_ba3bc/1
  Product_736ef/1 -> Add_ba3bc/2
  Product_12bd9/1 -> Divide_3c8e8/1
  Product_0e1d5/1 -> Divide_3c8e8/2
  Divide_3c8e8/1 -> Subtract_745a7/2
  Subtract_745a7/1 -> Product_86144/2

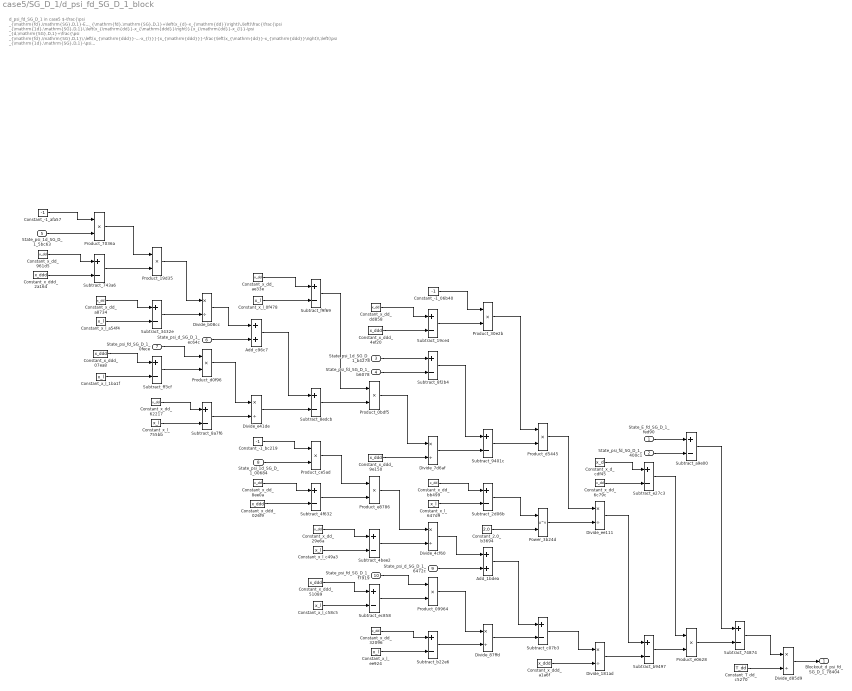
== system case5/SG_D_1/d_psi_fd_SG_D_1_block ==
  note: d_psi_fd_SG_D_1 in case5
      | $-\frac{\psi _{\mathrm{fd},\mathrm{SG},D,1}-E_{\mathrm{fd},\mathrm{SG},D,1}+\left(x_{d}-x_{\mathrm{dd}}\right)\,\left(\frac{\frac{\psi _{\mathrm{1d},\mathrm{SG},D,1}\,\left(x_{\mathrm{dd}}-x_{\mathrm{ddd}}\right)}{x_{\mathrm{dd}}-x_{l}}-\psi _{d,\mathrm{SG},D,1}+\frac{\psi _{\mathrm{fd},\mathrm{SG},D,1}\,\left(x_{\mathrm{ddd}}-x_{l}\right)}{x_{\mathrm{dd}}-x_{l}}}{x_{\mathrm{ddd}}}-\frac{\left(x_{\mathrm{dd}}-x_{\mathrm{ddd}}\right)\,\left(\psi _{\mathrm{1d},\mathrm{SG},D,1}-\psi _{\mathrm{fd},\mathrm{SG},D,1}+\frac{\left(x_{\mathrm{dd}}-x_{l}\right)\,\left(\frac{\psi _{\mathrm{1d},\mathrm{SG},D,1}\,\left(x_{\mathrm{dd}}-x_{\mathrm{ddd}}\right)}{x_{\mathrm{dd}}-x_{l}}-\psi _{d,\mathrm{SG},D,1}+\frac{\psi _{\mathrm{fd},\mathrm{SG},D,1}\,\left(x_{\mathrm{ddd}}-x_{l}\right)}{x_{\mathrm{dd}}-x_{l}}\right)}{x_{\mathrm{ddd}}}\right)}{{\left(x_{\mathrm{dd}}-x_{l}\right)}^2}\right)}{T_{\mathrm{dd}}}$
      | Automatically generated on 2025-10-31 19:09:51 .
  State_E_fd_SG_D_1_fed90 : Inport
  State_psi_fd_SG_D_1_400c1 : Inport  Port=2
  State_psi_1d_SG_D_1_b4278 : Inport  Port=3
  State_psi_fd_SG_D_1_b6078 : Inport  Port=4
  State_psi_1d_SG_D_1_5bc63 : Inport  Port=5
  State_psi_d_SG_D_1_ec64c : Inport  Port=6
  State_psi_fd_SG_D_1_0fece : Inport  Port=7
  State_psi_1d_SG_D_1_00684 : Inport  Port=8
  State_psi_d_SG_D_1_6472c : Inport  Port=9
  State_psi_fd_SG_D_1_f7919 : Inport  Port=10
  Add_1bdea : Sum
  Add_c96c7 : Sum
  Constant_-1_06b40 : Constant  Value=-1
  Constant_-1_afa57 : Constant  Value=-1
  Constant_-1_bc219 : Constant  Value=-1
  Constant_2.0_b3694 : Constant  Value=2.0
  Constant_T_dd_c5270 : Constant  Value=T_dd
  Constant_x_d_cdf45 : Constant  Value=x_d
  Constant_x_dd_29e6a : Constant  Value=x_dd
  Constant_x_dd_32096 : Constant  Value=x_dd
  Constant_x_dd_62217 : Constant  Value=x_dd
  Constant_x_dd_6c79c : Constant  Value=x_dd
  Constant_x_dd_8ee0a : Constant  Value=x_dd
  Constant_x_dd_961d5 : Constant  Value=x_dd
  Constant_x_dd_a8734 : Constant  Value=x_dd
  Constant_x_dd_ae33e : Constant  Value=x_dd
  Constant_x_dd_bb499 : Constant  Value=x_dd
  Constant_x_dd_dd858 : Constant  Value=x_dd
  Constant_x_ddd_026f9 : Constant  Value=x_ddd
  Constant_x_ddd_07ea8 : Constant  Value=x_ddd
  Constant_x_ddd_2a164 : Constant  Value=x_ddd
  Constant_x_ddd_4ef20 : Constant  Value=x_ddd
  Constant_x_ddd_51089 : Constant  Value=x_ddd
  Constant_x_ddd_9e150 : Constant  Value=x_ddd
  Constant_x_ddd_a1a6f : Constant  Value=x_ddd
  Constant_x_l_0f478 : Constant  Value=x_l
  Constant_x_l_1ba1f : Constant  Value=x_l
  Constant_x_l_647d9 : Constant  Value=x_l
  Constant_x_l_755bb : Constant  Value=x_l
  Constant_x_l_a54f4 : Constant  Value=x_l
  Constant_x_l_c49a3 : Constant  Value=x_l
  Constant_x_l_c58c5 : Constant  Value=x_l
  Constant_x_l_ee924 : Constant  Value=x_l
  Divide_181ad : Product  Inputs=*/
  Divide_4cf60 : Product  Inputs=*/
  Divide_7d6af : Product  Inputs=*/
  Divide_87ffd : Product  Inputs=*/
  Divide_b08cc : Product  Inputs=*/
  Divide_d85d9 : Product  Inputs=*/
  Divide_e41de : Product  Inputs=*/
  Divide_ee111 : Product  Inputs=*/
  Power_3b24d : Math  Operator=pow
  Product_09964 : Product
  Product_0bdf5 : Product
  Product_19d35 : Product
  Product_30e2b : Product
  Product_7036a : Product
  Product_ce5ad : Product
  Product_d0f96 : Product
  Product_d5445 : Product
  Product_e0628 : Product
  Product_e8786 : Product
  Subtract_19ce4 : Sum  Inputs=+-
  Subtract_2d06b : Sum  Inputs=+-
  Subtract_3432e : Sum  Inputs=+-
  Subtract_4bee2 : Sum  Inputs=+-
  Subtract_4f632 : Sum  Inputs=+-
  Subtract_743a6 : Sum  Inputs=+-
  Subtract_74874 : Sum  Inputs=+-
  Subtract_8a7f6 : Sum  Inputs=+-
  Subtract_8edcb : Sum  Inputs=+-
  Subtract_8f2b4 : Sum  Inputs=+-
  Subtract_9401c : Sum  Inputs=+-
  Subtract_a9e00 : Sum  Inputs=+-
  Subtract_b22e6 : Sum  Inputs=+-
  Subtract_b9497 : Sum  Inputs=+-
  Subtract_c07b3 : Sum  Inputs=+-
  Subtract_e27c3 : Sum  Inputs=+-
  Subtract_ec858 : Sum  Inputs=+-
  Subtract_f9f69 : Sum  Inputs=+-
  Subtract_ff3cf : Sum  Inputs=+-
  Blockout_d_psi_fd_SG_D_1_78404 : Outport
  wires:
  State_psi_d_SG_D_1_ec64c/1 -> Add_c96c7/2
  Constant_x_dd_a8734/1 -> Subtract_3432e/1
  Product_19d35/1 -> Divide_b08cc/1
  Subtract_743a6/1 -> Product_19d35/2
  Subtract_8edcb/1 -> Product_0bdf5/2
  Product_7036a/1 -> Product_19d35/1
  Constant_x_dd_961d5/1 -> Subtract_743a6/1
  Constant_x_l_0f478/1 -> Subtract_f9f69/2
  Constant_-1_afa57/1 -> Product_7036a/1
  Subtract_f9f69/1 -> Product_0bdf5/1
  Constant_x_l_a54f4/1 -> Subtract_3432e/2
  Constant_x_ddd_2a164/1 -> Subtract_743a6/2
  State_psi_1d_SG_D_1_5bc63/1 -> Product_7036a/2
  Constant_x_ddd_07ea8/1 -> Subtract_ff3cf/1
  Constant_x_l_1ba1f/1 -> Subtract_ff3cf/2
  State_E_fd_SG_D_1_fed90/1 -> Subtract_a9e00/1
  Divide_b08cc/1 -> Add_c96c7/1
  Subtract_3432e/1 -> Divide_b08cc/2
  State_psi_fd_SG_D_1_0fece/1 -> Product_d0f96/1
  Constant_x_ddd_9e150/1 -> Divide_7d6af/2
  Subtract_ff3cf/1 -> Product_d0f96/2
  Constant_x_dd_62217/1 -> Subtract_8a7f6/1
  Constant_x_dd_bb499/1 -> Subtract_2d06b/1
  State_psi_fd_SG_D_1_400c1/1 -> Subtract_a9e00/2
  Constant_x_l_755bb/1 -> Subtract_8a7f6/2
  Product_d0f96/1 -> Divide_e41de/1
  Constant_-1_06b40/1 -> Product_30e2b/1
  Subtract_8a7f6/1 -> Divide_e41de/2
  Constant_x_dd_ae33e/1 -> Subtract_f9f69/1
  Add_c96c7/1 -> Subtract_8edcb/1
  Constant_x_l_647d9/1 -> Subtract_2d06b/2
  Divide_e41de/1 -> Subtract_8edcb/2
  Divide_ee111/1 -> Subtract_b9497/1
  Constant_-1_bc219/1 -> Product_ce5ad/1
  State_psi_1d_SG_D_1_00684/1 -> Product_ce5ad/2
  Constant_x_dd_8ee0a/1 -> Subtract_4f632/1
  Subtract_19ce4/1 -> Product_30e2b/2
  Constant_x_ddd_026f9/1 -> Subtract_4f632/2
  Product_ce5ad/1 -> Product_e8786/1
  Constant_2.0_b3694/1 -> Power_3b24d/2
  Product_e8786/1 -> Divide_4cf60/1
  Subtract_b9497/1 -> Product_e0628/2
  Subtract_4f632/1 -> Product_e8786/2
  State_psi_d_SG_D_1_6472c/1 -> Add_1bdea/2
  Constant_x_dd_29e6a/1 -> Subtract_4bee2/1
  Constant_x_l_c49a3/1 -> Subtract_4bee2/2
  Constant_x_dd_dd858/1 -> Subtract_19ce4/1
  Divide_7d6af/1 -> Subtract_9401c/2
  Constant_x_ddd_51089/1 -> Subtract_ec858/1
  Constant_x_ddd_4ef20/1 -> Subtract_19ce4/2
  Constant_x_l_c58c5/1 -> Subtract_ec858/2
  Subtract_ec858/1 -> Product_09964/2
  State_psi_1d_SG_D_1_b4278/1 -> Subtract_8f2b4/1
  Product_09964/1 -> Divide_87ffd/1
  State_psi_fd_SG_D_1_b6078/1 -> Subtract_8f2b4/2
  State_psi_fd_SG_D_1_f7919/1 -> Product_09964/1
  Product_0bdf5/1 -> Divide_7d6af/1
  Divide_4cf60/1 -> Add_1bdea/1
  Subtract_4bee2/1 -> Divide_4cf60/2
  Constant_x_dd_32096/1 -> Subtract_b22e6/1
  Constant_x_l_ee924/1 -> Subtract_b22e6/2
  Divide_87ffd/1 -> Subtract_c07b3/2
  Subtract_8f2b4/1 -> Subtract_9401c/1
  Subtract_b22e6/1 -> Divide_87ffd/2
  Subtract_9401c/1 -> Product_d5445/2
  Product_30e2b/1 -> Product_d5445/1
  Subtract_2d06b/1 -> Power_3b24d/1
  Add_1bdea/1 -> Subtract_c07b3/1
  Product_d5445/1 -> Divide_ee111/1
  Power_3b24d/1 -> Divide_ee111/2
  Subtract_c07b3/1 -> Divide_181ad/1
  Constant_x_ddd_a1a6f/1 -> Divide_181ad/2
  Constant_x_d_cdf45/1 -> Subtract_e27c3/1
  Constant_x_dd_6c79c/1 -> Subtract_e27c3/2
  Divide_181ad/1 -> Subtract_b9497/2
  Subtract_e27c3/1 -> Product_e0628/1
  Subtract_a9e00/1 -> Subtract_74874/1
  Product_e0628/1 -> Subtract_74874/2
  Subtract_74874/1 -> Divide_d85d9/1
  Constant_T_dd_c5270/1 -> Divide_d85d9/2
  Divide_d85d9/1 -> Blockout_d_psi_fd_SG_D_1_78404/1

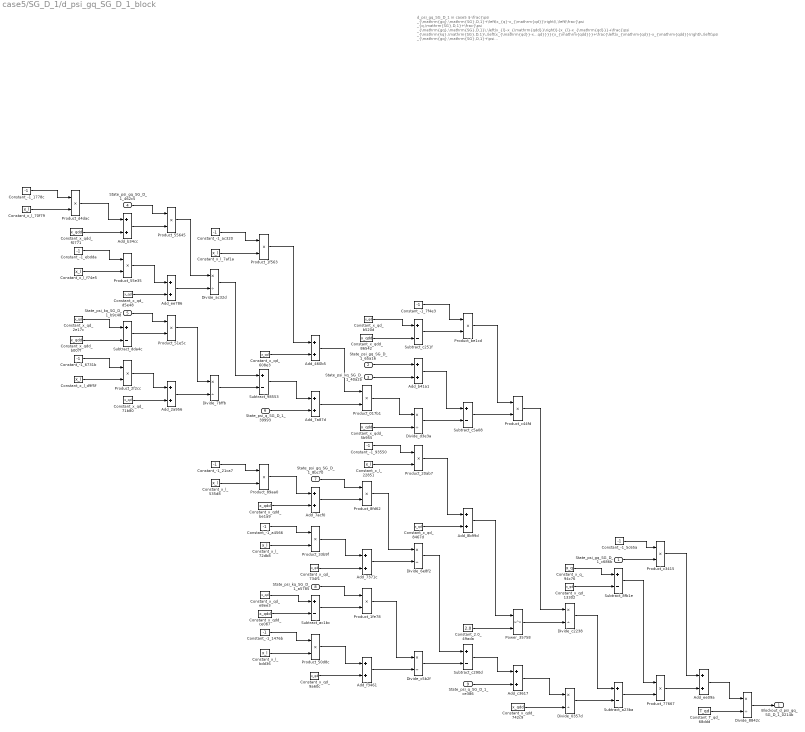
== system case5/SG_D_1/d_psi_gq_SG_D_1_block ==
  note: d_psi_gq_SG_D_1 in case5
      | $-\frac{\psi _{\mathrm{gq},\mathrm{SG},D,1}+\left(x_{q}-x_{\mathrm{qd}}\right)\,\left(\frac{\psi _{q,\mathrm{SG},D,1}+\frac{\psi _{\mathrm{gq},\mathrm{SG},D,1}\,\left(x_{l}-x_{\mathrm{qdd}}\right)}{x_{l}-x_{\mathrm{qd}}}+\frac{\psi _{\mathrm{kq},\mathrm{SG},D,1}\,\left(x_{\mathrm{qd}}-x_{\mathrm{qdd}}\right)}{x_{l}-x_{\mathrm{qd}}}}{x_{\mathrm{qdd}}}+\frac{\left(x_{\mathrm{qd}}-x_{\mathrm{qdd}}\right)\,\left(\psi _{\mathrm{gq},\mathrm{SG},D,1}+\psi _{\mathrm{kq},\mathrm{SG},D,1}+\frac{\left(x_{l}-x_{\mathrm{qd}}\right)\,\left(\psi _{q,\mathrm{SG},D,1}+\frac{\psi _{\mathrm{gq},\mathrm{SG},D,1}\,\left(x_{l}-x_{\mathrm{qdd}}\right)}{x_{l}-x_{\mathrm{qd}}}+\frac{\psi _{\mathrm{kq},\mathrm{SG},D,1}\,\left(x_{\mathrm{qd}}-x_{\mathrm{qdd}}\right)}{x_{l}-x_{\mathrm{qd}}}\right)}{x_{\mathrm{qdd}}}\right)}{{\left(x_{l}-x_{\mathrm{qd}}\right)}^2}\right)}{T_{\mathrm{qd}}}$
      | Automatically generated on 2025-10-31 19:10:00 .
  State_psi_gq_SG_D_1_c686b : Inport
  State_psi_gq_SG_D_1_65a16 : Inport  Port=2
  State_psi_kq_SG_D_1_40a2b : Inport  Port=3
  State_psi_gq_SG_D_1_462c5 : Inport  Port=4
  State_psi_kq_SG_D_1_b9c48 : Inport  Port=5
  State_psi_q_SG_D_1_39993 : Inport  Port=6
  State_psi_gq_SG_D_1_8bc70 : Inport  Port=7
  State_psi_kq_SG_D_1_a5785 : Inport  Port=8
  State_psi_q_SG_D_1_ce386 : Inport  Port=9
  Add_2a956 : Sum
  Add_460b5 : Sum
  Add_7371c : Sum
  Add_7a87d : Sum
  Add_7acf0 : Sum
  Add_8b99d : Sum
  Add_b34cc : Sum
  Add_b41a1 : Sum
  Add_c3617 : Sum
  Add_ee09a : Sum
  Add_ee786 : Sum
  Add_f3461 : Sum
  Constant_-1_1476b : Constant  Value=-1
  Constant_-1_1778c : Constant  Value=-1
  Constant_-1_21ca7 : Constant  Value=-1
  Constant_-1_5c65a : Constant  Value=-1
  Constant_-1_6731b : Constant  Value=-1
  Constant_-1_7f4e3 : Constant  Value=-1
  Constant_-1_93550 : Constant  Value=-1
  Constant_-1_a4566 : Constant  Value=-1
  Constant_-1_ac320 : Constant  Value=-1
  Constant_-1_ebdda : Constant  Value=-1
  Constant_2.0_49ada : Constant  Value=2.0
  Constant_T_qd_68ddd : Constant  Value=T_qd
  Constant_x_l_22851 : Constant  Value=x_l
  Constant_x_l_535d8 : Constant  Value=x_l
  Constant_x_l_70f79 : Constant  Value=x_l
  Constant_x_l_72db8 : Constant  Value=x_l
  Constant_x_l_7af1a : Constant  Value=x_l
  Constant_x_l_bdd36 : Constant  Value=x_l
  Constant_x_l_d9f5f : Constant  Value=x_l
  Constant_x_l_f74e5 : Constant  Value=x_l
  Constant_x_q_94c76 : Constant  Value=x_q
  Constant_x_qd_13302 : Constant  Value=x_qd
  Constant_x_qd_2e17c : Constant  Value=x_qd
  Constant_x_qd_608e3 : Constant  Value=x_qd
  Constant_x_qd_71b80 : Constant  Value=x_qd
  Constant_x_qd_734f1 : Constant  Value=x_qd
  Constant_x_qd_8467d : Constant  Value=x_qd
  Constant_x_qd_9a60c : Constant  Value=x_qd
  Constant_x_qd_b520d : Constant  Value=x_qd
  Constant_x_qd_d5e48 : Constant  Value=x_qd
  Constant_x_qd_e8ee3 : Constant  Value=x_qd
  Constant_x_qdd_5b955 : Constant  Value=x_qdd
  Constant_x_qdd_742c9 : Constant  Value=x_qdd
  Constant_x_qdd_86542 : Constant  Value=x_qdd
  Constant_x_qdd_b007f : Constant  Value=x_qdd
  Constant_x_qdd_be1a9 : Constant  Value=x_qdd
  Constant_x_qdd_ce0b7 : Constant  Value=x_qdd
  Constant_x_qdd_f0771 : Constant  Value=x_qdd
  Divide_0357d : Product  Inputs=*/
  Divide_6e8f2 : Product  Inputs=*/
  Divide_7bffb : Product  Inputs=*/
  Divide_8842c : Product  Inputs=*/
  Divide_ac32d : Product  Inputs=*/
  Divide_c2238 : Product  Inputs=*/
  Divide_c5b2f : Product  Inputs=*/
  Divide_d3e3a : Product  Inputs=*/
  Power_35758 : Math  Operator=pow
  Product_017b1 : Product
  Product_1f563 : Product
  Product_1fe78 : Product
  Product_20ab7 : Product
  Product_2f2cc : Product
  Product_33b9f : Product
  Product_50d8c : Product
  Product_51e5c : Product
  Product_55645 : Product
  Product_55e35 : Product
  Product_77667 : Product
  Product_89aa0 : Product
  Product_8fd62 : Product
  Product_be1cd : Product
  Product_c3415 : Product
  Product_c44fd : Product
  Product_d4dac : Product
  Subtract_8fb1e : Sum  Inputs=+-
  Subtract_98553 : Sum  Inputs=+-
  Subtract_a23ba : Sum  Inputs=+-
  Subtract_ac1bc : Sum  Inputs=+-
  Subtract_c251f : Sum  Inputs=+-
  Subtract_c290d : Sum  Inputs=+-
  Subtract_c5a08 : Sum  Inputs=+-
  Subtract_dda4c : Sum  Inputs=+-
  Blockout_d_psi_gq_SG_D_1_0214b : Outport
  wires:
  State_psi_gq_SG_D_1_462c5/1 -> Product_55645/1
  Constant_-1_ebdda/1 -> Product_55e35/1
  Divide_ac32d/1 -> Subtract_98553/1
  Add_ee786/1 -> Divide_ac32d/2
  Product_d4dac/1 -> Add_b34cc/1
  Constant_x_qd_608e3/1 -> Add_460b5/2
  Constant_-1_1778c/1 -> Product_d4dac/1
  Constant_x_qdd_f0771/1 -> Add_b34cc/2
  Constant_x_l_f74e5/1 -> Product_55e35/2
  Constant_x_l_70f79/1 -> Product_d4dac/2
  Constant_-1_6731b/1 -> Product_2f2cc/1
  Constant_x_qd_2e17c/1 -> Subtract_dda4c/1
  Constant_x_qdd_5b955/1 -> Divide_d3e3a/2
  Constant_x_l_d9f5f/1 -> Product_2f2cc/2
  Constant_x_qdd_b007f/1 -> Subtract_dda4c/2
  Subtract_98553/1 -> Add_7a87d/1
  Add_b34cc/1 -> Product_55645/2
  Product_55645/1 -> Divide_ac32d/1
  Product_55e35/1 -> Add_ee786/1
  Constant_x_qd_d5e48/1 -> Add_ee786/2
  State_psi_kq_SG_D_1_b9c48/1 -> Product_51e5c/1
  Product_2f2cc/1 -> Add_2a956/1
  Subtract_dda4c/1 -> Product_51e5c/2
  Constant_x_qd_71b80/1 -> Add_2a956/2
  Product_51e5c/1 -> Divide_7bffb/1
  Add_2a956/1 -> Divide_7bffb/2
  Constant_-1_7f4e3/1 -> Product_be1cd/1
  Constant_-1_ac320/1 -> Product_1f563/1
  Add_7371c/1 -> Divide_6e8f2/2
  Product_50d8c/1 -> Add_f3461/1
  Subtract_ac1bc/1 -> Product_1fe78/2
  Constant_x_l_7af1a/1 -> Product_1f563/2
  Divide_7bffb/1 -> Subtract_98553/2
  Subtract_8fb1e/1 -> Product_77667/1
  Constant_-1_93550/1 -> Product_20ab7/1
  Constant_-1_21ca7/1 -> Product_89aa0/1
  Constant_x_l_22851/1 -> Product_20ab7/2
  Constant_x_l_535d8/1 -> Product_89aa0/2
  Constant_x_qd_734f1/1 -> Add_7371c/2
  Product_1f563/1 -> Add_460b5/1
  State_psi_q_SG_D_1_39993/1 -> Add_7a87d/2
  Product_89aa0/1 -> Add_7acf0/1
  Constant_x_qdd_be1a9/1 -> Add_7acf0/2
  Constant_-1_a4566/1 -> Product_33b9f/1
  Constant_x_qd_9a60c/1 -> Add_f3461/2
  Add_460b5/1 -> Product_017b1/1
  Constant_x_l_72db8/1 -> Product_33b9f/2
  Constant_-1_1476b/1 -> Product_50d8c/1
  Constant_x_qd_e8ee3/1 -> Subtract_ac1bc/1
  Product_017b1/1 -> Divide_d3e3a/1
  Constant_x_l_bdd36/1 -> Product_50d8c/2
  Divide_c2238/1 -> Subtract_a23ba/1
  Constant_x_qdd_ce0b7/1 -> Subtract_ac1bc/2
  Add_7a87d/1 -> Product_017b1/2
  State_psi_gq_SG_D_1_8bc70/1 -> Product_8fd62/1
  Add_7acf0/1 -> Product_8fd62/2
  Product_33b9f/1 -> Add_7371c/1
  State_psi_kq_SG_D_1_a5785/1 -> Product_1fe78/1
  Add_f3461/1 -> Divide_c5b2f/2
  State_psi_gq_SG_D_1_65a16/1 -> Add_b41a1/1
  Constant_x_qd_b520d/1 -> Subtract_c251f/1
  Constant_x_qdd_86542/1 -> Subtract_c251f/2
  Product_1fe78/1 -> Divide_c5b2f/1
  State_psi_kq_SG_D_1_40a2b/1 -> Add_b41a1/2
  Product_8fd62/1 -> Divide_6e8f2/1
  Subtract_c251f/1 -> Product_be1cd/2
  Add_b41a1/1 -> Subtract_c5a08/1
  Divide_d3e3a/1 -> Subtract_c5a08/2
  Product_20ab7/1 -> Add_8b99d/1
  Constant_x_qd_8467d/1 -> Add_8b99d/2
  Divide_6e8f2/1 -> Subtract_c290d/1
  Divide_c5b2f/1 -> Subtract_c290d/2
  Product_be1cd/1 -> Product_c44fd/1
  Subtract_c5a08/1 -> Product_c44fd/2
  Add_8b99d/1 -> Power_35758/1
  Constant_2.0_49ada/1 -> Power_35758/2
  Subtract_c290d/1 -> Add_c3617/1
  State_psi_q_SG_D_1_ce386/1 -> Add_c3617/2
  Product_c44fd/1 -> Divide_c2238/1
  Power_35758/1 -> Divide_c2238/2
  Add_c3617/1 -> Divide_0357d/1
  Constant_x_qdd_742c9/1 -> Divide_0357d/2
  Constant_x_q_94c76/1 -> Subtract_8fb1e/1
  Constant_x_qd_13302/1 -> Subtract_8fb1e/2
  Divide_0357d/1 -> Subtract_a23ba/2
  Constant_-1_5c65a/1 -> Product_c3415/1
  State_psi_gq_SG_D_1_c686b/1 -> Product_c3415/2
  Subtract_a23ba/1 -> Product_77667/2
  Product_c3415/1 -> Add_ee09a/1
  Product_77667/1 -> Add_ee09a/2
  Add_ee09a/1 -> Divide_8842c/1
  Constant_T_qd_68ddd/1 -> Divide_8842c/2
  Divide_8842c/1 -> Blockout_d_psi_gq_SG_D_1_0214b/1
